simulink model "Problem10"  (R2020b)
settings: Solver=VariableStepAuto  StartTime=0.0  StopTime=10.0  RelTol=1e-3
model workspace (MAT data in the model file):
  Ia = Simulink.Parameter
  Ia.Value = [0 0 0 0 1]
  Ia.DataType = 'auto'
  Ia.Dimensions = [1 5]
  Vo = Simulink.Parameter
  Vo.Value = [0.2 0.4 0.6 0.8 1]
  Vo.DataType = 'auto'
  Vo.Dimensions = [1 5]
libraries: simulink x1
settings Model: Creator=Acer  LastModifiedBy=Acer

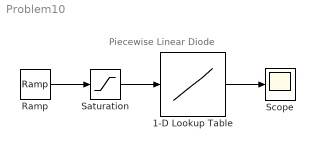
== system Problem10 ==
  note: Piecewise Linear Diode
  1-D Lookup Table : Lookup_n-D  NumberOfTableDimensions=1  BreakpointsForDimension1=Vo  Table=Ia  InternalRulePriority=Speed  RndMeth=Simplest  InputSameDT=on
  Ramp : simulink/Sources/Ramp  slope=1  start=0  InitialOutput=0
  Saturation : Saturate  UpperLimit=9  LowerLimit=0
  Scope : Scope
  wires:
  1-D Lookup Table/1 -> Scope/1
  Saturation/1 -> 1-D Lookup Table/1
  Ramp/1 -> Saturation/1
